simulink model "KPA_ALL"  (R2022b)
settings: Solver=FixedStepAuto  StartTime=0.0  StopTime=1  RelTol=1e-3
model workspace (MAT data in the model file):
  OutputBufferSize = 2
  OutputSampesPerSymbol = 4
  OutputSamplesPerSymbol = 4
  SNR = 16
  SampleTimeGenerator = 2.5e-06
undefined symbols (not defined in the file or in its folder): Add, DiscIntNeverNeededParam, magnitude, Shift
libraries: hdlsllib x16, simulink x5, commhdlcrc x3, commdigbbndpm3 x2, commfilt2 x2, commdigbbndam3 x2, commchan3 x1, commseqgen3 x1, commrandsrc3 x1, commsync2 x1, commsink2 x1, commutil2 x1
(part 2 of 2)

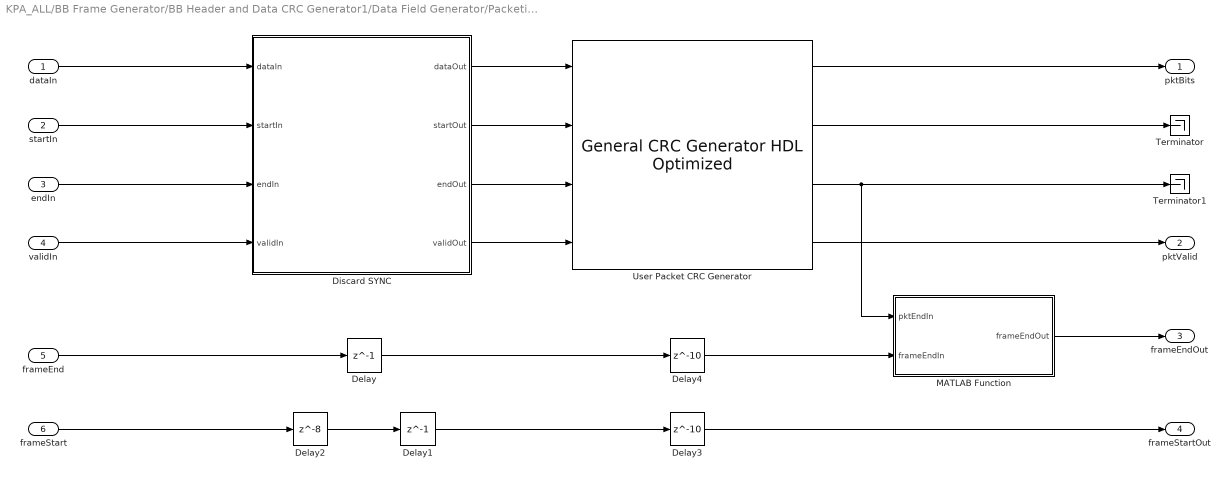
== system KPA_ALL/BB Frame Generator/BB Header and Data CRC Generator1/Data Field Generator/Packetized Streams ==
  dataIn : Inport
  startIn : Inport  Port=2
  endIn : Inport  Port=3
  validIn : Inport  Port=4
  frameEnd : Inport  Port=5
  frameStart : Inport  Port=6
  Delay : Delay  DelayLength=1
  Delay1 : Delay  DelayLength=1
  Delay2 : Delay  DelayLength=8
  Delay3 : Delay  DelayLength=10
  Delay4 : Delay  DelayLength=10
  Discard SYNC : MATLAB Function  TreatAsAtomicUnit=on
  MATLAB Function : MATLAB Function  TreatAsAtomicUnit=on
  Terminator : Terminator
  Terminator1 : Terminator
  User Packet CRC Generator : commhdlcrc/General CRC Generator HDL Optimized  Polynomial=[1 1 1 0 1 0 1 0 1]  InitialState=0  DirectMethod=off  ReflectInput=off  ReflectCRCChecksum=off  FinalXORValue=0  SimulateUsing=Code generation
  pktBits : Outport
  pktValid : Outport  Port=2
  frameEndOut : Outport  Port=3
  frameStartOut : Outport  Port=4
  wires:
  Discard SYNC/1(dataOut) -> User Packet CRC Generator/1
  MATLAB Function/1(frameEndOut) -> frameEndOut/1
  Delay2/1 -> Delay1/1
  Delay/1 -> Delay4/1
  validIn/1 -> Discard SYNC/4(validIn)
  dataIn/1 -> Discard SYNC/1(dataIn)
  Discard SYNC/4(validOut) -> User Packet CRC Generator/4
  User Packet CRC Generator/3 -> Terminator1/1, MATLAB Function/1(pktEndIn)
  User Packet CRC Generator/2 -> Terminator/1
  Discard SYNC/3(endOut) -> User Packet CRC Generator/3
  Discard SYNC/2(startOut) -> User Packet CRC Generator/2
  Delay1/1 -> Delay3/1
  User Packet CRC Generator/1 -> pktBits/1
  frameStart/1 -> Delay2/1
  frameEnd/1 -> Delay/1
  startIn/1 -> Discard SYNC/2(startIn)
  endIn/1 -> Discard SYNC/3(endIn)
  Delay3/1 -> frameStartOut/1
  User Packet CRC Generator/4 -> pktValid/1
  Delay4/1 -> MATLAB Function/2(frameEndIn)

== matlab function KPA_ALL/BB Frame Generator/BB Header and Data CRC Generator1/BB Header Generator/BB Header Packetizer ==
  data: startIn input; TSorGS input; dataOut output; startOut output; endOut output; validOut output; DFL input; UPL input; SYNC input; countOut output

function [dataOut,startOut,endOut,validOut,countOut] = BBHeaderCount(startIn,TSorGS,DFL,UPL,SYNC)
%#codegen

persistent count dataReg startReg endReg validReg;
   if isempty(count)
       count = fi(72,0,nextpow2(80),0,hdlfimath);
       dataReg = false;
       startReg = false;
       endReg = false;
       validReg = false;
   end

   dataOut = dataReg;
   startOut = startReg;
   endOut = endReg;
   validOut = validReg;
   countOut = count;
   
   dataReg = false;
   validReg = false;
   startReg = false;
   endReg = false;
   
   if startIn
       count(:) = 0;
   end
   
       if count < 72
           validReg = true;
           if count == 0
               dataReg = logical(bitget(TSorGS,2));       % MSB of TS/GS
               startReg = true;                           % start of header
           elseif count == 1
               dataReg = logical(bitget(TSorGS,1));       % LSB of TS/GS
           elseif (count == 2) || (count == 3)
               dataReg = true;                            % SIS/MIS, CCM/ACM
%            elseif (count >= 4) && (count <= 15)           % ISSYI, NPD, RO, MATTYPE-2
           elseif (count >= 16) && (count <= 31)
               dataReg = logical(bitget(UPL,uint8(32-count)));   % UPL
           elseif (count >= 32) && (count <= 47) % DFL
               dataReg = logical(bitget(DFL,uint8(48-count)));   % DFL
           elseif (count >= 48) && (count <= 55)          % SYNC
               dataReg = logical(bitget(SYNC,uint8(56-count)));
%            elseif (count >= 56) && (count <= 71)          % SYNCD
           elseif count == 71
               endReg = true;                             % end of header
           end
           count(:) = count + 1;
       else
           validReg = false;
       end
   

end

== matlab function KPA_ALL/BB Frame Generator/BB Header and Data CRC Generator/BB Header Generator/BB Header Packetizer ==
  data: startIn input; TSorGS input; dataOut output; startOut output; endOut output; validOut output; DFL input; UPL input; SYNC input; countOut output

function [dataOut,startOut,endOut,validOut,countOut] = BBHeaderCount(startIn,TSorGS,DFL,UPL,SYNC)
%#codegen

persistent count dataReg startReg endReg validReg;
   if isempty(count)
       count = fi(72,0,nextpow2(80),0,hdlfimath);
       dataReg = false;
       startReg = false;
       endReg = false;
       validReg = false;
   end

   dataOut = dataReg;
   startOut = startReg;
   endOut = endReg;
   validOut = validReg;
   countOut = count;
   
   dataReg = false;
   validReg = false;
   startReg = false;
   endReg = false;
   
   if startIn
       count(:) = 0;
   end
   
       if count < 72
           validReg = true;
           if count == 0
               dataReg = logical(bitget(TSorGS,2));       % MSB of TS/GS
               startReg = true;                           % start of header
           elseif count == 1
               dataReg = logical(bitget(TSorGS,1));       % LSB of TS/GS
           elseif (count == 2) || (count == 3)
               dataReg = true;                            % SIS/MIS, CCM/ACM
%            elseif (count >= 4) && (count <= 15)           % ISSYI, NPD, RO, MATTYPE-2
           elseif (count >= 16) && (count <= 31)
               dataReg = logical(bitget(UPL,uint8(32-count)));   % UPL
           elseif (count >= 32) && (count <= 47) % DFL
               dataReg = logical(bitget(DFL,uint8(48-count)));   % DFL
           elseif (count >= 48) && (count <= 55)          % SYNC
               dataReg = logical(bitget(SYNC,uint8(56-count)));
%            elseif (count >= 56) && (count <= 71)          % SYNCD
           elseif count == 71
               endReg = true;                             % end of header
           end
           count(:) = count + 1;
       else
           validReg = false;
       end
   

end

== matlab function KPA_ALL/BB Frame Generator/BB Header and Data CRC Generator1/Data Field Generator/Packetized Streams/Discard SYNC ==
  data: dataIn input; dataOut output; startIn input; endIn input; validIn input; startOut output; endOut output; validOut output
function [dataOut,startOut,endOut,validOut] = discardSYNC(dataIn,startIn,endIn,validIn)
%#codegen


persistent count dataReg validReg startReg endReg;
    if isempty(count)
        count = fi(0,0,4,0,hdlfimath);
        dataReg = cast(0,'like',dataIn);
        validReg = false;
        startReg = false;
        endReg = false;
    end

    dataOut = dataReg;
    validOut = validReg;
    startOut = startReg;
    endOut = endReg;

    if startIn
        count(:) = 0;
    end
 
    if validIn
        if (count < 8)
            startReg = false;
            validReg = false;
        elseif count == 8
            startReg = true;
            validReg = true;
        else
            startReg = false;
            validReg = true;
        end
        if count < 9
            count(:) = count + 1;
        end
    else
        validReg = false;
        startReg = false;
    end
    if validReg
        dataReg = dataIn;
        endReg = endIn;
    else
        dataReg(:) = 0;
        endReg = false;
    end

end

== matlab function KPA_ALL/BB Frame Generator/BB Header and Data CRC Generator1/Data Field Generator/Packetized Streams/MATLAB Function ==
  data: pktEndIn input; frameEndOut output; frameEndIn input
function frameEndOut = fcn(pktEndIn,frameEndIn)
%#codegen

    persistent frameEnded;
    if isempty(frameEnded)
        frameEnded = false;
    end

    if frameEndIn
        frameEnded = true;
    end

    if pktEndIn && frameEnded
        frameEndOut = true;
        frameEnded = false;
    else
        frameEndOut = false;
    end


end

== matlab function KPA_ALL/BB Frame Generator/BB Header and Data CRC Generator1/MATLAB Function ==
  data: validIn input; startIn input; endIn input; validAppend output; DFL input; endAppend output
function [validAppend,endAppend] = DFLLengthCounter(validIn,startIn,endIn,DFL)
%#codegen
   
   MAX_DFL = 58192-80; 
   persistent countDFL isEndReceived;
   if isempty(countDFL)
       countDFL = fi(0,0,nextpow2(MAX_DFL),0,hdlfimath);
       isEndReceived = false;
   end
   
   if startIn
       countDFL(:) = 0;
   end

   if isEndReceived
       validAppend = true;
       countDFL(:) = countDFL + 1;
   elseif validIn
       validAppend = false;
       countDFL(:) = countDFL + 1;
   else
       validAppend = false;
   end
   
   if countDFL > DFL
       validAppend = false;
   end
   if DFL ~= 0
       if countDFL >= DFL
           endAppend = isEndReceived;
           isEndReceived = false;
       else
           endAppend = false;
       end
   else
       endAppend = false;
   end

   if endIn
       isEndReceived = true;
   end
end

== matlab function KPA_ALL/BB Frame Generator/BB Header and Data CRC Generator1/MATLAB Function1 ==
  data: u input; y output
function y = monostable(u)
%#codegen

   persistent count countActive;
   if isempty(count)
       count = fi(0,0,nextpow2(80),0,hdlfimath);
       countActive = false;
   end

   y = countActive;
    
   if count == 79
       countActive = false;
       count(:) = 0;
   end
   if countActive
       count(:) = count + 1;
   end
   if u 
       countActive = true;
   end

end

== matlab function KPA_ALL/BB Frame Generator/Data Store FIFO/MATLAB Function ==
  data: startIn input; validOut output; DFL input; endOut output
function [validOut,endOut] = DFLLengthCounter(startIn,DFL)
%#codegen
   
   persistent countDFL countActive;
   if isempty(countDFL)
       countDFL = cast(0,'like',DFL);
       countActive = false;
   end

   validOut = countActive;
   endOut = countActive && (countDFL == DFL);

   
   if (DFL ~= 0) && (countDFL == DFL)
       countActive = false;
   end



   if startIn
       countDFL(:) = 0;
       countActive = true;
   end

   if countActive
       countDFL(:) = countDFL + 1;
   end



end

== matlab function KPA_ALL/BB Frame Generator/Data Store FIFO/RAM status ==
  data: full output; ncount output; wr input; empty output; rd input
function [full,ncount,empty] = fcn(wr,rd)
%#codegen
     
    WL = 7;
    persistent count;
    if isempty(count)
        count = fi(0,0,WL+1,0,hdlfimath);
    end

    empty = (count == 0);
    full = (count > 2^WL-1);
    ncount = count;

    if wr
        count(:) = count + 1;
    end
    if rd
        count(:) = count - 1;
    end

end
